simulink model "EV_Modeling"  (R2024b)
settings: Solver=FixedStepAuto  StartTime=0.0  StopTime=inf  FixedStep=0.1  RelTol=1e-3
values from neighbouring files (symbols this model uses):
  battery_SOC_resistance = battery_SOC(:,3)    [EV_Truck.m]
  battery_SOC_SOC = battery_SOC(:,1)    [EV_Truck.m]
  battery_SOC_voltage = battery_SOC(:,2)    [EV_Truck.m]
  motor_efficiency_efficiency = table2array(motor_efficiency(2:height(motor_efficiency),2:width(motor_efficiency)))    [EV_Truck.m]
  motor_efficiency_RPM = table2array(motor_efficiency(2:height(motor_efficiency),1))    [EV_Truck.m]
  motor_efficiency_torque = transpose(motor_efficiency_torque)    [EV_Truck.m]
  motor_RPM_torque = table2array(motor_torque(1:6,1))    [EV_Truck.m]
  motor_torque_RPM = table2array(motor_torque(1:6,2))    [EV_Truck.m]
undefined symbols (not defined in the file or in its folder): battery_builder_rtmsupport, DiscIntNeverNeededParam, gcbh, recurrentNet
libraries: simulink x8, fl_lib x6, nesl_utility x6, dlutilitylib x4, dlsequencelib x4, Batteries_lib x3, dlconvfclib x3, mpcadaslib x2, slpidlib x2, dlactivationlib x2, simulink_extras x1
(part 3 of 3)

== matlab function EV_Modeling/FV1/ACC system/MATLAB Function ==
  data: accel input; acceleration output
function acceleration  = fcn(accel)

if accel > 0 
    acceleration = (accel * 100)/0.15;
elseif accel < 0 
    acceleration = (accel * 100)/0.33;
else
    acceleration = 0; % accel이 0이거나 NaN일 경우에도 대응
end

== matlab function EV_Modeling/FV1/Drag coefficient ==
  data: IVD input; C_drag output
function C_drag = fcn(IVD)
a = -0.4629;
b = -0.068;
c = 0.6441;

C_drag = a * exp(b * (IVD-8)) + c;
